simulink model "Fig270"  (R2014b)
settings: Solver=ode3  StartTime=0.0  StopTime=1  FixedStep=2e-5  RelTol=1e-5
libraries: dsparch4 x2, commrandsrc2 x1
settings Model: Creator=Dennis Silage  LastModifiedBy=Silage
settings DataIOCC: SignalLoggingSaveFormat=ModelDataLogs
settings OptimizationCC: ExpressionDepthLimit=2147483647  InitFltsAndDblsToZero=on
settings DebuggingCC: UnderspecifiedInitializationDetection=Classic  MergeDetectMultiDrivingBlocksExec=none  SolverPrmCheckMsg=none  FcnCallInpInsideContextMsg=UseLocalSettings  StateNameClashWarn=warning
settings GRTTargetCC: CombineOutputUpdateFcns=off  GRTInterface=on

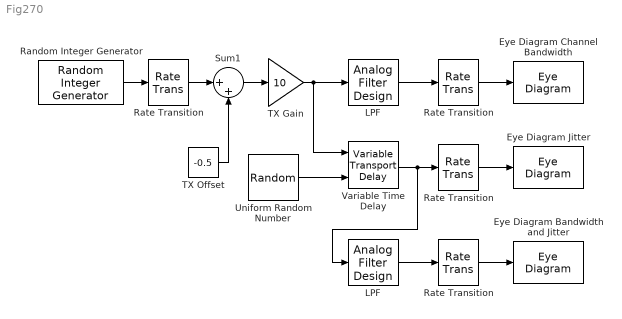
== system Fig270 ==
  Eye Diagram Bandwidth and Jitter : EyeDiagram  Tag=EyeDiagram
  Eye Diagram Channel Bandwidth : EyeDiagram  Tag=EyeDiagram
  Eye Diagram Jitter : EyeDiagram  Tag=EyeDiagram
  LPF : dsparch4/Analog Filter Design  method=Chebyshev I  filttype=Lowpass  N=9  Wlo=2*pi*1200  Whi=80  Rp=0.1  Rs=40
  "LPF " : dsparch4/Analog Filter Design  method=Chebyshev I  filttype=Lowpass  N=9  Wlo=2*pi*1200  Whi=80  Rp=0.1  Rs=40
  Random Integer Generator : commrandsrc2/Random Integer Generator  mul=2  seed=randseed  Ts=1e-3  frameBased=off  sampPerFrame=50  orient=on  outDataType=double
  "Rate Transition " : RateTransition  OutPortSampleTime=2e-5
  "Rate Transition " : RateTransition  OutPortSampleTime=2e-5
  Rate Transition : RateTransition  OutPortSampleTime=2e-5
  "Rate Transition " : RateTransition  OutPortSampleTime=2e-5
  Sum1 : Sum  Inputs=|++
  TX Gain : Gain  Gain=10
  TX Offset : Constant  Value=-0.5
  Uniform Random Number : UniformRandomNumber  Minimum=0.00002  Maximum=0.0005  SampleTime=0
  Variable Time Delay : VariableTransportDelay  MaximumDelay=.0025  ZeroDelay=on  TransDelayFeedthrough=on
  wires:
  TX Gain/1 -> LPF/1, Variable Time Delay/1
  Random Integer Generator/1 -> Rate Transition/1
  Rate Transition/1 -> Sum1/1
  Sum1/1 -> TX Gain/1
  TX Offset/1 -> Sum1/2
  "Rate Transition "/1 -> Eye Diagram Channel Bandwidth/1
  LPF/1 -> "Rate Transition "/1
  Variable Time Delay/1 -> "LPF "/1, "Rate Transition "/1
  "Rate Transition "/1 -> Eye Diagram Jitter/1
  Uniform Random Number/1 -> Variable Time Delay/2
  "Rate Transition "/1 -> Eye Diagram Bandwidth and Jitter/1
  "LPF "/1 -> "Rate Transition "/1
